simulink model "SystemBlockDiagram"  (R2020a)
settings: Solver=VariableStepAuto  StartTime=0.0  StopTime=10.0  RelTol=1e-3
settings Model: DataDictionary=RobotDD.sldd  OrderedModelArguments=off  Creator=Sony  LastModifiedBy=Sony

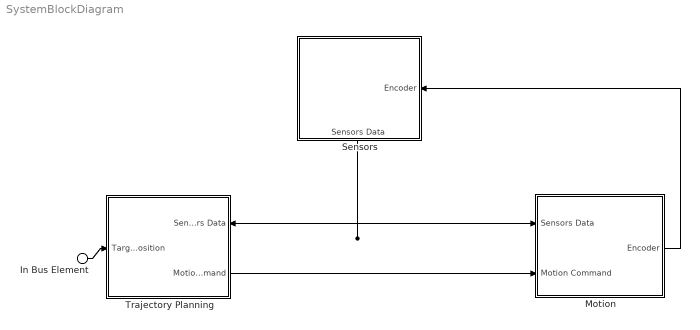
== system SystemBlockDiagram ==
  In Bus Element : Inport  PortName=Target Position
  Motion : Subsystem
      settings: PortSchema="{\"entries\":[{\"content\":{\"headerSize\":26,\"margin\":15,\"minimumSpacing\":25,\"sides\":[{\"content\":{\"connectorIds\":[\"In1\",\"In2\"]},\"type\":\"ConnectorPlacement.EquallySpacedRectSide\",\"uuid\":\"a373f431-dc92-4815-b0cc-0f6ebc017e21\"},{\"content\":{\"connectorIds\":[\"Out1\"],\"side\":\"RIGHT\"},\"type\":\"ConnectorPlacement.EquallySpacedRectSide\",\"uuid\":\"7d2ad539-b7f2-4a3f-b190-c92a0c72bdef\"},{\"content\":{\"connectorIds\":[],\"side\":\"TOP\"},\"type\":\"ConnectorPlacement.EquallySpacedRectSide\",\"uuid\":\"a9aec8db-ef01-47e6-840b-bfb59ce405a8\"}]},\"type\":\"ConnectorPlacement.EquallySpacedConnector\",\"uuid\":\"ba89a8aa-546b-4b6e-ba99-aa9ff0eba9d8\"}],\"packageUris\":[\"http://schema.mathworks.com/mf0/Connector/19700101\"],\"version\":\"1.0\"}"
  Sensors : Subsystem
      settings: PortSchema="{\"entries\":[{\"content\":{\"headerSize\":26,\"margin\":15,\"minimumSpacing\":25,\"sides\":[{\"content\":{\"connectorIds\":[]},\"type\":\"ConnectorPlacement.EquallySpacedRectSide\",\"uuid\":\"a373f431-dc92-4815-b0cc-0f6ebc017e21\"},{\"content\":{\"connectorIds\":[\"In1\"],\"side\":\"RIGHT\"},\"type\":\"ConnectorPlacement.EquallySpacedRectSide\",\"uuid\":\"7d2ad539-b7f2-4a3f-b190-c92a0c72bdef\"},{\"content\":{\"connectorIds\":[],\"side\":\"TOP\"},\"type\":\"ConnectorPlacement.EquallySpacedRectSide\",\"uuid\":\"a9aec8db-ef01-47e6-840b-bfb59ce405a8\"},{\"content\":{\"connectorIds\":[\"Out1\"],\"side\":\"BOTTOM\"},\"type\":\"ConnectorPlacement.EquallySpacedRectSide\",\"uuid\":\"aa5e38e1-9d2c-44e3-83b3-72e7a74461d8\"}]},\"type\":\"ConnectorPlacement.EquallySpacedConnector\",\"uuid\":\"ba89a8aa-546b-4b6e-ba99-aa9ff0eba9d8\"}],\"packageUris\":[\"http://schema.mathworks.com/mf0/Connector/19700101\"],\"version\":\"1.0\"}"
  Trajectory Planning : Subsystem
      settings: PortSchema="{\"entries\":[{\"content\":{\"headerSize\":26,\"margin\":15,\"minimumSpacing\":25,\"sides\":[{\"content\":{\"connectorIds\":[\"In1\"]},\"type\":\"ConnectorPlacement.EquallySpacedRectSide\",\"uuid\":\"a373f431-dc92-4815-b0cc-0f6ebc017e21\"},{\"content\":{\"connectorIds\":[\"In2\",\"Out1\"],\"side\":\"RIGHT\"},\"type\":\"ConnectorPlacement.EquallySpacedRectSide\",\"uuid\":\"7d2ad539-b7f2-4a3f-b190-c92a0c72bdef\"},{\"content\":{\"connectorIds\":[],\"side\":\"TOP\"},\"type\":\"ConnectorPlacement.EquallySpacedRectSide\",\"uuid\":\"a9aec8db-ef01-47e6-840b-bfb59ce405a8\"}]},\"type\":\"ConnectorPlacement.EquallySpacedConnector\",\"uuid\":\"ba89a8aa-546b-4b6e-ba99-aa9ff0eba9d8\"}],\"packageUris\":[\"http://schema.mathworks.com/mf0/Connector/19700101\"],\"version\":\"1.0\"}"
  wires:
  Sensors/1(Sensors Data) -> Trajectory Planning/2(Sensors Data), Motion/1(Sensors Data)
  Trajectory Planning/1(Motion Command) -> Motion/2(Motion Command)
  Motion/1(Encoder) -> Sensors/1(Encoder)
  In Bus Element/1 -> Trajectory Planning/1(Target Position)

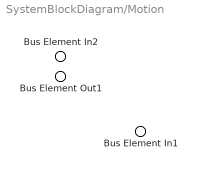
== system SystemBlockDiagram/Motion ==
  Bus Element In1 : Inport  PortName=Sensors Data
  Bus Element In2 : Inport  Port=2  PortName=Motion Command
  Bus Element Out1 : Outport  PortName=Encoder

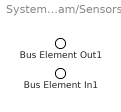
== system SystemBlockDiagram/Sensors ==
  Bus Element In1 : Inport  PortName=Encoder
  Bus Element Out1 : Outport  PortName=Sensors Data

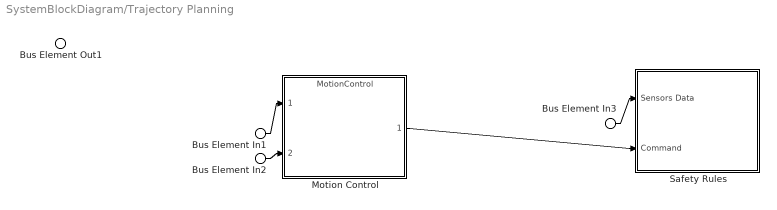
== system SystemBlockDiagram/Trajectory Planning ==
  Bus Element In2 : Inport  PortName=Target Position
  Bus Element In1 : Inport  Port=2  PortName=Sensors Data
  Bus Element In3 : Inport  Port=2  PortName=Sensors Data
  Motion Control : ModelReference  ModelNameDialog=MotionControl  SimulationMode=Normal  ModelReferenceVersion=1.4
      settings: PortSchema="{\"entries\":[{\"content\":{\"headerSize\":38,\"margin\":15,\"minimumSpacing\":25,\"sides\":[{\"content\":{\"connectorIds\":[\"In1\",\"In2\"]},\"type\":\"ConnectorPlacement.EquallySpacedRectSide\",\"uuid\":\"a373f431-dc92-4815-b0cc-0f6ebc017e21\"},{\"content\":{\"connectorIds\":[\"Out1\"],\"side\":\"RIGHT\"},\"type\":\"ConnectorPlacement.EquallySpacedRectSide\",\"uuid\":\"7d2ad539-b7f2-4a3f-b190-c92a0c72bdef\"},{\"content\":{\"connectorIds\":[],\"side\":\"TOP\"},\"type\":\"ConnectorPlacement.EquallySpacedRectSide\",\"uuid\":\"a9aec8db-ef01-47e6-840b-bfb59ce405a8\"}]},\"type\":\"ConnectorPlacement.EquallySpacedConnector\",\"uuid\":\"ba89a8aa-546b-4b6e-ba99-aa9ff0eba9d8\"}],\"packageUris\":[\"http://schema.mathworks.com/mf0/Connector/19700101\"],\"version\":\"1.0\"}"
  Safety Rules : Subsystem
      settings: PortSchema="{\"entries\":[{\"content\":{\"headerSize\":26,\"margin\":15,\"minimumSpacing\":25,\"sides\":[{\"content\":{\"connectorIds\":[\"In1\",\"In2\"]},\"type\":\"ConnectorPlacement.EquallySpacedRectSide\",\"uuid\":\"a373f431-dc92-4815-b0cc-0f6ebc017e21\"},{\"content\":{\"connectorIds\":[],\"side\":\"RIGHT\"},\"type\":\"ConnectorPlacement.EquallySpacedRectSide\",\"uuid\":\"7d2ad539-b7f2-4a3f-b190-c92a0c72bdef\"},{\"content\":{\"connectorIds\":[],\"side\":\"TOP\"},\"type\":\"ConnectorPlacement.EquallySpacedRectSide\",\"uuid\":\"a9aec8db-ef01-47e6-840b-bfb59ce405a8\"}]},\"type\":\"ConnectorPlacement.EquallySpacedConnector\",\"uuid\":\"ba89a8aa-546b-4b6e-ba99-aa9ff0eba9d8\"}],\"packageUris\":[\"http://schema.mathworks.com/mf0/Connector/19700101\"],\"version\":\"1.0\"}"
  Bus Element Out1 : Outport  PortName=Motion Command
  wires:
  Bus Element In3/1 -> Safety Rules/1(Sensors Data)
  Bus Element In1/1 -> Motion Control/1
  Bus Element In2/1 -> Motion Control/2
  Motion Control/1 -> Safety Rules/2(Command)

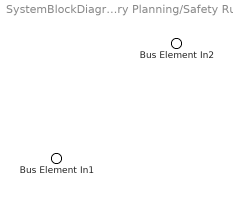
== system SystemBlockDiagram/Trajectory Planning/Safety Rules ==
  Bus Element In2 : Inport  PortName=Sensors Data
  Bus Element In1 : Inport  Port=2  PortName=Command
